simulink model "ar_lht_hw"  (R2018a)
settings: Solver=VariableStepAuto  StartTime=0.0  StopTime=ts*3+maxRho*2*T*3  RelTol=1e-3  EnableMultiTasking=on
PreLoadFcn:
  | currentDir  = pwd;
  | filesepIdx   = strfind(currentDir, filesep);
  | newDir = currentDir(1:filesepIdx(end)-7);
  | 
  | addpath([newDir, '\scripts']);
InitFcn:
  | setup;
  | pre_processing;
StopFcn:
  | post_processing;
  | imtool(O);
values from neighbouring files (symbols this model uses):
  deltaTheta = 1    [setup.m]
  fps = f/((height)*(width))    (= 1475.01627604)    [setup.m]
  height = 256    [setup.m]
  K = (maxTheta + deltaTheta)/R    (= 45)    [setup.m]
  maxRho = ceil(sqrt((height/2)^2+(width/2)^2))    [setup.m]
  maxTheta = 179    [setup.m]
  R = 4    [setup.m]
  T = 1/f    (= 6.89655172414e-09)    [setup.m]
  width = 384    [setup.m]
libraries: xbsIndex_r4 x336, hdlsllib x6, visionhdlutilities x2, visionhdlio x2, simulink x1, dspswit3 x1, visionsources x1
(part 2 of 2)

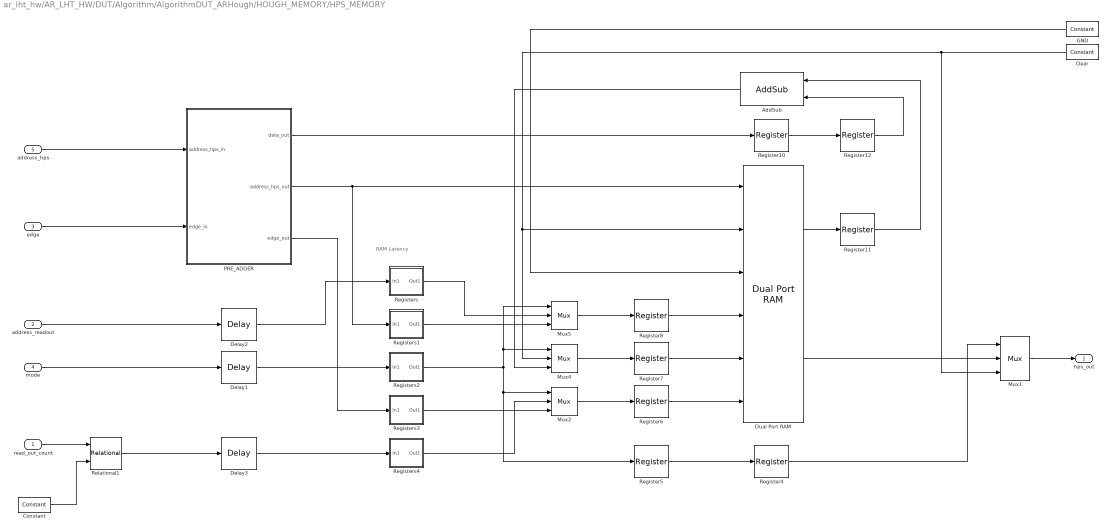
== system ar_lht_hw/AR_LHT_HW/DUT/Algorithm/AlgorithmDUT_ARHough/HOUGH_MEMORY/HPS_MEMORY ==
  note: RAM Latency
  read_out_count : Inport
  address_readout : Inport  Port=2
  edge : Inport  Port=3
  mode : Inport  Port=4
  address_hps : Inport  Port=5
  AddSub : xbsIndex_r4/AddSub  mode=Addition  use_carryin=off  use_carryout=off  en=off  latency=1  precision=User Defined  arith_type=Unsigned  n_bits=ceil(log2(maxRho*2))  bin_pt=0  quantization=Truncate  overflow=Wrap  use_behavioral_HDL=off  hw_selection=Fabric  pipelined=off  dbl_ovrd=off  block_type=addsub
  Clear : xbsIndex_r4/Constant  const=0  gui_display_data_type=Fixed-point  arith_type=Unsigned  n_bits=9  bin_pt=0  preci_type=Single  exp_width=8  frac_width=24  explicit_period=on  period=T  equ=P=C  opselect=C  inp2=PCIN>>17  opr=+  inp1=P  carry=CIN  dbl_ovrd=off  block_type=constant
  Constant : xbsIndex_r4/Constant  const=R-1  gui_display_data_type=Fixed-point  arith_type=Unsigned  n_bits=ceil(log2(R))  bin_pt=0  preci_type=Single  exp_width=8  frac_width=24  explicit_period=on  period=T  equ=P=C  opselect=C  inp2=PCIN>>17  opr=+  inp1=P  carry=CIN  dbl_ovrd=off  block_type=constant
  Delay1 : xbsIndex_r4/Delay  rst=off  infoeditControl=Selection of Reset will increase slice count due to use of real FFs and instead of SRLs  en=off  latency=7  reg_retiming=off  dbl_ovrd=off  block_type=delay
  Delay2 : xbsIndex_r4/Delay  rst=off  infoeditControl=Selection of Reset will increase slice count due to use of real FFs and instead of SRLs  en=off  latency=7  reg_retiming=off  dbl_ovrd=off  block_type=delay
  Delay3 : xbsIndex_r4/Delay  rst=off  infoeditControl=Selection of Reset will increase slice count due to use of real FFs and instead of SRLs  en=off  latency=7  reg_retiming=off  dbl_ovrd=off  block_type=delay
  Dual Port RAM : xbsIndex_r4/Dual Port RAM  depth=K*maxRho*2  initVector=0  distributed_mem=Block RAM  init_a=0  init_b=0  rst_a=off  rst_b=off  en_a=off  en_b=off  latency=1  write_mode_A=Read Before Write  write_mode_B=Read Before Write  optimize=Area  dbl_ovrd=off  block_type=dpram
  GND : xbsIndex_r4/Constant  const=0  gui_display_data_type=Boolean  arith_type=Boolean  n_bits=18  bin_pt=0  preci_type=Single  exp_width=8  frac_width=24  explicit_period=on  period=T  equ=P=C  opselect=C  inp2=PCIN>>17  opr=+  inp1=P  carry=CIN  dbl_ovrd=off  block_type=constant
  Mux1 : xbsIndex_r4/Mux  inputs=2  en=off  latency=1  precision=Full  arith_type=Unsigned  n_bits=16  bin_pt=14  quantization=Truncate  overflow=Wrap  dbl_ovrd=off  block_type=mux
  Mux2 : xbsIndex_r4/Mux  inputs=2  en=off  latency=0  precision=Full  arith_type=Unsigned  n_bits=16  bin_pt=14  quantization=Truncate  overflow=Wrap  dbl_ovrd=off  block_type=mux
  Mux4 : xbsIndex_r4/Mux  inputs=2  en=off  latency=0  precision=Full  arith_type=Unsigned  n_bits=16  bin_pt=14  quantization=Truncate  overflow=Wrap  dbl_ovrd=off  block_type=mux
  Mux5 : xbsIndex_r4/Mux  inputs=2  en=off  latency=0  precision=Full  arith_type=Unsigned  n_bits=16  bin_pt=14  quantization=Truncate  overflow=Wrap  dbl_ovrd=off  block_type=mux
  PRE_ADDER : Subsystem
  Register{4..8,10..12} (8 alike) : xbsIndex_r4/Register  init=0  rst=off  en=off  dbl_ovrd=off  block_type=register
  Registers : Subsystem
  Registers1 : Subsystem
  Registers2 : Subsystem
  Registers3 : Subsystem
  Registers4 : Subsystem
  Relational1 : xbsIndex_r4/Relational  mode=a=b  op_type=Bool  en=off  latency=0  dbl_ovrd=off  block_type=relational
  hps_out : Outport
  wires:
  Register12/1 -> AddSub/2
  Register11/1 -> AddSub/1
  Delay3/1 -> Registers4/1(In1)
  Delay1/1 -> Registers2/1(In1)
  Delay2/1 -> Registers/1(In1)
  Register10/1 -> Register12/1
  Registers1/1(Out1) -> Mux5/3
  Registers/1(Out1) -> Mux5/2
  Registers2/1(Out1) -> Mux4/1, Mux5/1, Mux2/1, Register5/1
  Registers3/1(Out1) -> Mux2/3
  Registers4/1(Out1) -> Mux2/2
  address_readout/1 -> Delay2/1
  Relational1/1 -> Delay3/1
  mode/1 -> Delay1/1
  AddSub/1 -> Mux4/3
  PRE_ADDER/1(data_out) -> Register10/1
  Dual Port RAM/1 -> Register11/1
  PRE_ADDER/3(edge_out) -> Registers3/1(In1)
  PRE_ADDER/2(address_hps_out) -> Dual Port RAM/1, Registers1/1(In1)
  edge/1 -> PRE_ADDER/2(edge_in)
  address_hps/1 -> PRE_ADDER/1(address_hps_in)
  read_out_count/1 -> Relational1/1
  GND/1 -> Dual Port RAM/3
  Register8/1 -> Dual Port RAM/4
  Mux5/1 -> Register8/1
  Mux4/1 -> Register7/1
  Mux2/1 -> Register6/1
  Register7/1 -> Dual Port RAM/5
  Register6/1 -> Dual Port RAM/6
  Register5/1 -> Register4/1
  Dual Port RAM/2 -> Mux1/2
  Clear/1 -> Mux1/3, Mux4/2, Dual Port RAM/2
  Mux1/1 -> hps_out/1
  Constant/1 -> Relational1/2
  Register4/1 -> Mux1/1

== system ar_lht_hw/AR_LHT_HW/DUT/Algorithm/AlgorithmDUT_ARHough/HOUGH_MEMORY/RBM_MEMORY ==
  edge : Inport
  mode : Inport  Port=2
  address_rbm : Inport  Port=3
  readout_rbm : Inport  Port=4
  ClearData : xbsIndex_r4/Constant  const=0  gui_display_data_type=Boolean  arith_type=Boolean  n_bits=9  bin_pt=0  preci_type=Single  exp_width=8  frac_width=24  explicit_period=on  period=T  equ=P=C  opselect=C  inp2=PCIN>>17  opr=+  inp1=P  carry=CIN  dbl_ovrd=off  block_type=constant
  Delay4 : xbsIndex_r4/Delay  rst=off  infoeditControl=Selection of Reset will increase slice count due to use of real FFs and instead of SRLs  en=off  latency=10  reg_retiming=off  dbl_ovrd=off  block_type=delay
  Mux1 : xbsIndex_r4/Mux  inputs=2  en=off  latency=1  precision=User Defined  arith_type=Unsigned  n_bits=1  bin_pt=0  quantization=Truncate  overflow=Wrap  dbl_ovrd=off  block_type=mux
  Mux4 : xbsIndex_r4/Mux  inputs=2  en=off  latency=0  precision=Full  arith_type=Unsigned  n_bits=16  bin_pt=14  quantization=Truncate  overflow=Wrap  dbl_ovrd=off  block_type=mux
  Mux6 : xbsIndex_r4/Mux  inputs=2  en=off  latency=0  precision=Full  arith_type=Unsigned  n_bits=16  bin_pt=14  quantization=Truncate  overflow=Wrap  dbl_ovrd=off  block_type=mux
  Mux7 : xbsIndex_r4/Mux  inputs=2  en=off  latency=0  precision=Full  arith_type=Unsigned  n_bits=16  bin_pt=14  quantization=Truncate  overflow=Wrap  dbl_ovrd=off  block_type=mux
  Register{1..5} (5 alike) : xbsIndex_r4/Register  init=0  rst=off  en=off  dbl_ovrd=off  block_type=register
  Single Port RAM : xbsIndex_r4/Single Port RAM  depth=(maxTheta+deltaTheta)*maxRho*2  initVector=0  distributed_mem=Block RAM  write_mode=Read Before Write  rst=off  init_reg=0  en=off  latency=1  optimize=Area  dbl_ovrd=off  block_type=spram
  vcc : xbsIndex_r4/Constant  const=1  gui_display_data_type=Boolean  arith_type=Boolean  n_bits=9  bin_pt=0  preci_type=Single  exp_width=8  frac_width=24  explicit_period=on  period=T  equ=P=C  opselect=C  inp2=PCIN>>17  opr=+  inp1=P  carry=CIN  dbl_ovrd=off  block_type=constant
  rbm_out : Outport
  wires:
  Delay4/1 -> rbm_out/1
  Register5/1 -> Single Port RAM/1
  Register4/1 -> Single Port RAM/2
  Register3/1 -> Single Port RAM/3
  Register2/1 -> Register1/1
  Register1/1 -> Mux1/1
  mode/1 -> Mux7/1, Mux6/1, Mux4/1, Register2/1
  Single Port RAM/1 -> Mux1/2
  Mux1/1 -> Delay4/1
  vcc/1 -> Mux7/2, Mux6/3
  edge/1 -> Mux7/3
  ClearData/1 -> Mux1/3, Mux6/2
  Mux6/1 -> Register4/1
  Mux7/1 -> Register3/1
  Mux4/1 -> Register5/1
  address_rbm/1 -> Mux4/3
  readout_rbm/1 -> Mux4/2

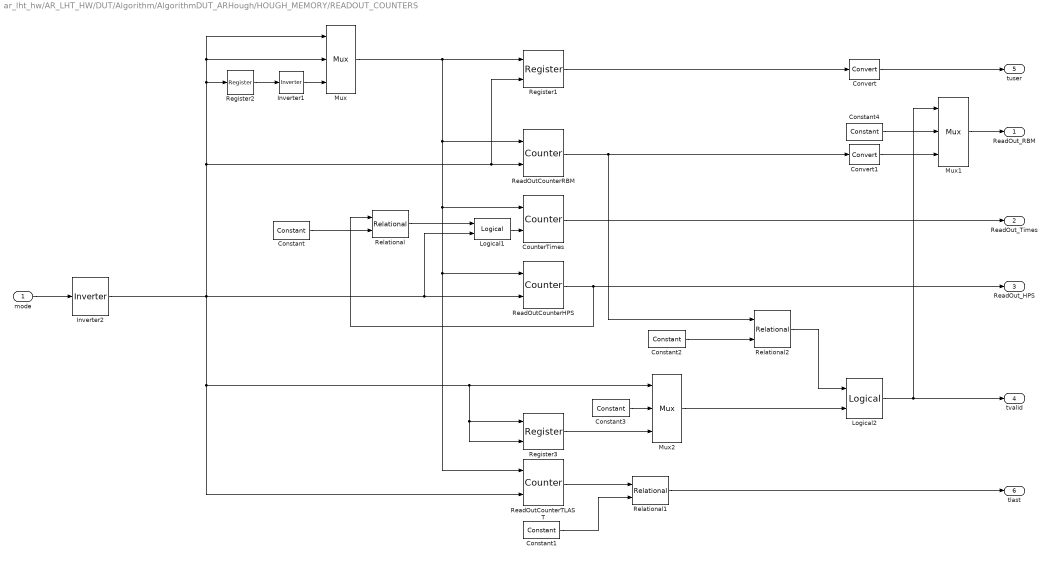
== system ar_lht_hw/AR_LHT_HW/DUT/Algorithm/AlgorithmDUT_ARHough/HOUGH_MEMORY/READOUT_COUNTERS ==
  mode : Inport
  Constant : xbsIndex_r4/Constant  const=K*maxRho*2-2  gui_display_data_type=Fixed-point  arith_type=Unsigned  n_bits=ceil(log2(K*maxRho*2-2))  bin_pt=0  preci_type=Single  exp_width=8  frac_width=24  explicit_period=on  period=T  equ=P=C  opselect=C  inp2=PCIN>>17  opr=+  inp1=P  carry=CIN  dbl_ovrd=off  block_type=constant
  Constant1 : xbsIndex_r4/Constant  const=2*maxRho-1  gui_display_data_type=Fixed-point  arith_type=Unsigned  n_bits=ceil(log2(2*maxRho-1))  bin_pt=0  preci_type=Single  exp_width=8  frac_width=24  explicit_period=on  period=T  equ=P=C  opselect=C  inp2=PCIN>>17  opr=+  inp1=P  carry=CIN  dbl_ovrd=off  block_type=constant
  Constant2 : xbsIndex_r4/Constant  const=(maxTheta+deltaTheta)*maxRho*2-1  gui_display_data_type=Fixed-point  arith_type=Unsigned  n_bits=ceil(log2((maxTheta+deltaTheta)*maxRho*2-1))  bin_pt=0  preci_type=Single  exp_width=8  frac_width=24  explicit_period=on  period=T  equ=P=C  opselect=C  inp2=PCIN>>17  opr=+  inp1=P  carry=CIN  dbl_ovrd=off  block_type=constant
  Constant3 : xbsIndex_r4/Constant  const=0  gui_display_data_type=Boolean  arith_type=Boolean  n_bits=16  bin_pt=14  preci_type=Single  exp_width=8  frac_width=24  explicit_period=on  period=T  equ=P=C  opselect=C  inp2=PCIN>>17  opr=+  inp1=P  carry=CIN  dbl_ovrd=off  block_type=constant
  Constant4 : xbsIndex_r4/Constant  const=0  gui_display_data_type=Fixed-point  arith_type=Unsigned  n_bits=ceil(log2((maxTheta+deltaTheta)*maxRho*2-1))  bin_pt=0  preci_type=Single  exp_width=8  frac_width=24  explicit_period=on  period=T  equ=P=C  opselect=C  inp2=PCIN>>17  opr=+  inp1=P  carry=CIN  dbl_ovrd=off  block_type=constant
  Convert : xbsIndex_r4/Convert  gui_display_data_type=Fixed-point  arith_type=Unsigned  n_bits=1  bin_pt=0  float_type=Single  exp_bits=8  fraction_bits=24  quantization=Truncate  overflow=Wrap  en=off  latency=0  pipeline=off  dbl_ovrd=off  block_type=convert
  Convert1 : xbsIndex_r4/Convert  gui_display_data_type=Fixed-point  arith_type=Unsigned  n_bits=ceil(log2((maxTheta+deltaTheta)*maxRho*2-1))  bin_pt=0  float_type=Single  exp_bits=8  fraction_bits=24  quantization=Truncate  overflow=Wrap  en=off  latency=0  pipeline=off  dbl_ovrd=off  block_type=convert
  CounterTimes : xbsIndex_r4/Counter  cnt_type=Count Limited  cnt_to=R-1  operation=Up  start_count=0  cnt_by_val=1  arith_type=Unsigned  n_bits=ceil(log2(R))  bin_pt=0  load_pin=off  rst=on  en=on  explicit_period=on  period=T  use_behavioral_HDL=on  implementation=Fabric  dbl_ovrd=off  block_type=counter
  Inverter1 : xbsIndex_r4/Inverter  en=off  latency=0  dbl_ovrd=off  block_type=inv
  Inverter2 : xbsIndex_r4/Inverter  en=off  latency=0  dbl_ovrd=off  block_type=inv
  Logical1 : xbsIndex_r4/Logical  logical_function=AND  inputs=2  en=off  latency=0  precision=Full  arith_type=Unsigned  n_bits=16  bin_pt=0  align_bp=on  dbl_ovrd=off  block_type=logical
  Logical2 : xbsIndex_r4/Logical  logical_function=AND  inputs=2  en=off  latency=0  precision=Full  arith_type=Unsigned  n_bits=16  bin_pt=0  align_bp=on  dbl_ovrd=off  block_type=logical
  Mux : xbsIndex_r4/Mux  inputs=2  en=off  latency=0  precision=Full  arith_type=Unsigned  n_bits=16  bin_pt=14  quantization=Truncate  overflow=Wrap  dbl_ovrd=off  block_type=mux
  Mux1 : xbsIndex_r4/Mux  inputs=2  en=off  latency=0  precision=Full  arith_type=Unsigned  n_bits=16  bin_pt=14  quantization=Truncate  overflow=Wrap  dbl_ovrd=off  block_type=mux
  Mux2 : xbsIndex_r4/Mux  inputs=2  en=off  latency=0  precision=Full  arith_type=Unsigned  n_bits=16  bin_pt=14  quantization=Truncate  overflow=Wrap  dbl_ovrd=off  block_type=mux
  ReadOutCounterHPS : xbsIndex_r4/Counter  cnt_type=Count Limited  cnt_to=K*maxRho*2-1  operation=Up  start_count=0  cnt_by_val=1  arith_type=Unsigned  n_bits=ceil(log2(K*maxRho*2-1))  bin_pt=0  load_pin=off  rst=on  en=on  explicit_period=on  period=T  use_behavioral_HDL=on  implementation=Fabric  dbl_ovrd=off  block_type=counter
  ReadOutCounterRBM : xbsIndex_r4/Counter  cnt_type=Free Running  cnt_to=(maxTheta+deltaTheta)*maxRho*2-1  operation=Up  start_count=0  cnt_by_val=1  arith_type=Unsigned  n_bits=32  bin_pt=0  load_pin=off  rst=on  en=on  explicit_period=on  period=T  use_behavioral_HDL=on  implementation=Fabric  dbl_ovrd=off  block_type=counter
  ReadOutCounterTLAST : xbsIndex_r4/Counter  cnt_type=Count Limited  cnt_to=2*maxRho - 1  operation=Up  start_count=0  cnt_by_val=1  arith_type=Unsigned  n_bits=ceil(log2(2*maxRho-1))  bin_pt=0  load_pin=off  rst=on  en=on  explicit_period=on  period=T  use_behavioral_HDL=on  implementation=Fabric  dbl_ovrd=off  block_type=counter
  Register1 : xbsIndex_r4/Register  init=0  rst=off  en=on  dbl_ovrd=off  block_type=register
  Register2 : xbsIndex_r4/Register  init=0  rst=off  en=off  dbl_ovrd=off  block_type=register
  Register3 : xbsIndex_r4/Register  init=0  rst=off  en=on  dbl_ovrd=off  block_type=register
  Relational : xbsIndex_r4/Relational  mode=a=b  op_type=Bool  en=off  latency=1  dbl_ovrd=off  block_type=relational
  Relational1 : xbsIndex_r4/Relational  mode=a=b  op_type=Bool  en=off  latency=0  dbl_ovrd=off  block_type=relational
  Relational2 : xbsIndex_r4/Relational  mode=a<=b  op_type=Bool  en=off  latency=0  dbl_ovrd=off  block_type=relational
  ReadOut_RBM : Outport
  ReadOut_Times : Outport  Port=2
  ReadOut_HPS : Outport  Port=3
  tvalid : Outport  Port=4
  tuser : Outport  Port=5
  tlast : Outport  Port=6
  wires:
  Logical2/1 -> Mux1/1, tvalid/1
  Constant4/1 -> Mux1/2
  Convert1/1 -> Mux1/3
  Mux1/1 -> ReadOut_RBM/1
  Constant3/1 -> Mux2/2
  Inverter2/1 -> Register2/1, Mux/2, Mux/1, ReadOutCounterRBM/2, Register1/2, ReadOutCounterHPS/2, Logical1/2, Mux2/1, Register3/1, Register3/2, ReadOutCounterTLAST/2
  Mux2/1 -> Logical2/2
  Register3/1 -> Mux2/3
  Relational2/1 -> Logical2/1
  Register1/1 -> Convert/1
  Mux/1 -> ReadOutCounterRBM/1, CounterTimes/1, ReadOutCounterHPS/1, ReadOutCounterTLAST/1, Register1/1
  Constant2/1 -> Relational2/2
  Convert/1 -> tuser/1
  Constant1/1 -> Relational1/2
  ReadOutCounterTLAST/1 -> Relational1/1
  Relational1/1 -> tlast/1
  Inverter1/1 -> Mux/3
  Register2/1 -> Inverter1/1
  mode/1 -> Inverter2/1
  ReadOutCounterHPS/1 -> Relational/1, ReadOut_HPS/1
  CounterTimes/1 -> ReadOut_Times/1
  ReadOutCounterRBM/1 -> Convert1/1, Relational2/1
  Constant/1 -> Relational/2
  Logical1/1 -> CounterTimes/2
  Relational/1 -> Logical1/1

== system ar_lht_hw/AR_LHT_HW/DUT/Algorithm/AlgorithmDUT_Open/MorphoOpen/POSITION_CALCULATOR ==
  tuser_in : Inport
  tvalid_in : Inport  Port=2
  Constant1 : xbsIndex_r4/Constant  const=width/2  gui_display_data_type=Fixed-point  arith_type=Unsigned  n_bits=ceil(log2(width/2))+1  bin_pt=0  preci_type=Single  exp_width=8  frac_width=24  explicit_period=on  period=T  equ=P=C  opselect=C  inp2=PCIN>>17  opr=+  inp1=P  carry=CIN  dbl_ovrd=off  block_type=constant
  Constant2 : xbsIndex_r4/Constant  const=height/2  gui_display_data_type=Fixed-point  arith_type=Unsigned  n_bits=ceil(log2(height/2))+1  bin_pt=0  preci_type=Single  exp_width=8  frac_width=24  explicit_period=on  period=T  equ=P=C  opselect=C  inp2=PCIN>>17  opr=+  inp1=P  carry=CIN  dbl_ovrd=off  block_type=constant
  Convert : xbsIndex_r4/Convert  gui_display_data_type=Boolean  arith_type=Boolean  n_bits=16  bin_pt=14  float_type=Single  exp_bits=8  fraction_bits=24  quantization=Truncate  overflow=Wrap  en=off  latency=0  pipeline=off  dbl_ovrd=off  block_type=convert
  Logical : xbsIndex_r4/Logical  logical_function=AND  inputs=2  en=off  latency=0  precision=Full  arith_type=Unsigned  n_bits=16  bin_pt=0  align_bp=on  dbl_ovrd=off  block_type=logical
  Logical1 : xbsIndex_r4/Logical  logical_function=OR  inputs=2  en=off  latency=0  precision=Full  arith_type=Unsigned  n_bits=16  bin_pt=0  align_bp=on  dbl_ovrd=off  block_type=logical
  Logical2 : xbsIndex_r4/Logical  logical_function=AND  inputs=2  en=off  latency=0  precision=Full  arith_type=Unsigned  n_bits=16  bin_pt=0  align_bp=on  dbl_ovrd=off  block_type=logical
  Relational : xbsIndex_r4/Relational  mode=a=b  op_type=Bool  en=off  latency=0  dbl_ovrd=off  block_type=relational
  Relational1 : xbsIndex_r4/Relational  mode=a=b  op_type=Bool  en=off  latency=0  dbl_ovrd=off  block_type=relational
  x_counter : xbsIndex_r4/Counter  cnt_type=Count Limited  cnt_to=width/2  operation=Up  start_count=-width/2+1  cnt_by_val=1  arith_type="Signed  (2's comp)"  n_bits=ceil(log2(width))+1  bin_pt=0  load_pin=off  rst=on  en=on  explicit_period=on  period=T  use_behavioral_HDL=on  implementation=Fabric  dbl_ovrd=off  block_type=counter
  y_counter : xbsIndex_r4/Counter  cnt_type=Count Limited  cnt_to=height/2  operation=Up  start_count=-height/2+1  cnt_by_val=1  arith_type="Signed  (2's comp)"  n_bits=ceil(log2(height))+1  bin_pt=0  load_pin=off  rst=on  en=on  explicit_period=on  period=T  use_behavioral_HDL=on  implementation=Fabric  dbl_ovrd=off  block_type=counter
  x_coordinate : Outport
  y_coordinate : Outport  Port=2
  wires:
  Relational1/1 -> Logical2/2
  Constant2/1 -> Relational1/2
  Logical2/1 -> Logical1/2
  Convert/1 -> Logical1/1
  Logical1/1 -> x_counter/1, y_counter/1
  y_counter/1 -> y_coordinate/1, Relational1/1
  Constant1/1 -> Relational/2
  x_counter/1 -> x_coordinate/1, Relational/1
  tuser_in/1 -> Convert/1
  Logical/1 -> y_counter/2
  Relational/1 -> Logical/1, Logical2/1
  tvalid_in/1 -> Logical/2, x_counter/2

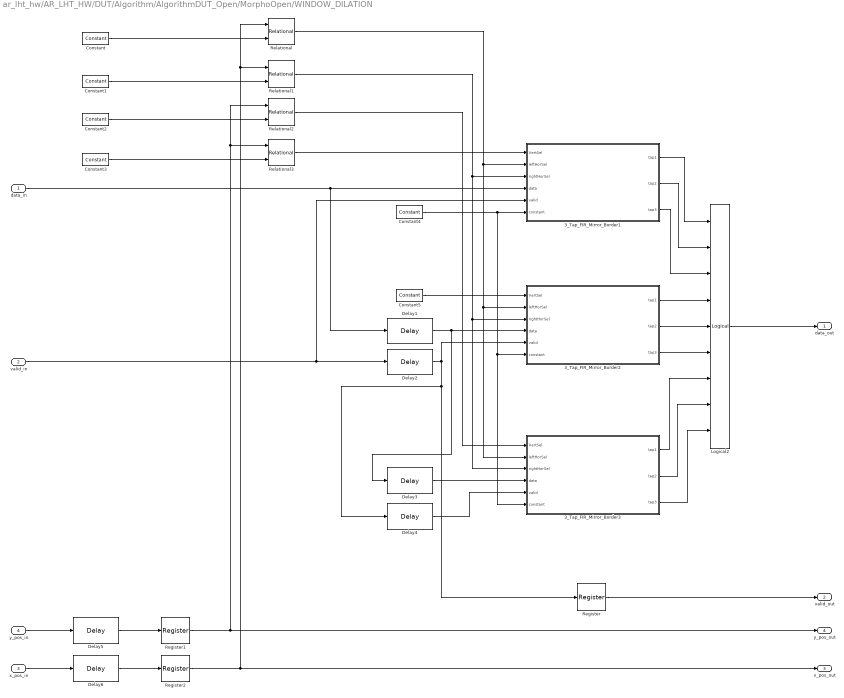
== system ar_lht_hw/AR_LHT_HW/DUT/Algorithm/AlgorithmDUT_Open/MorphoOpen/WINDOW_DILATION ==
  data_in : Inport
  valid_in : Inport  Port=2
  x_pos_in : Inport  Port=3
  y_pos_in : Inport  Port=4
  3_Tap_FIR_Mirror_Border1 : Subsystem
  3_Tap_FIR_Mirror_Border2 : Subsystem
  3_Tap_FIR_Mirror_Border3 : Subsystem
  Constant : xbsIndex_r4/Constant  const=-width/2+1  gui_display_data_type=Fixed-point  arith_type=Signed (2's comp)  n_bits=ceil(log2(width))+1  bin_pt=0  preci_type=Single  exp_width=8  frac_width=24  explicit_period=on  period=T  equ=P=C  opselect=C  inp2=PCIN>>17  opr=+  inp1=P  carry=CIN  dbl_ovrd=off  block_type=constant
  Constant1 : xbsIndex_r4/Constant  const=width/2  gui_display_data_type=Fixed-point  arith_type=Unsigned  n_bits=ceil(log2(width/2))+1  bin_pt=0  preci_type=Single  exp_width=8  frac_width=24  explicit_period=on  period=T  equ=P=C  opselect=C  inp2=PCIN>>17  opr=+  inp1=P  carry=CIN  dbl_ovrd=off  block_type=constant
  Constant2 : xbsIndex_r4/Constant  const=-height/2+1  gui_display_data_type=Fixed-point  arith_type=Signed (2's comp)  n_bits=ceil(log2(height))+1  bin_pt=0  preci_type=Single  exp_width=8  frac_width=24  explicit_period=on  period=T  equ=P=C  opselect=C  inp2=PCIN>>17  opr=+  inp1=P  carry=CIN  dbl_ovrd=off  block_type=constant
  Constant3 : xbsIndex_r4/Constant  const=height/2  gui_display_data_type=Fixed-point  arith_type=Unsigned  n_bits=ceil(log2(height/2))+1  bin_pt=0  preci_type=Single  exp_width=8  frac_width=24  explicit_period=on  period=T  equ=P=C  opselect=C  inp2=PCIN>>17  opr=+  inp1=P  carry=CIN  dbl_ovrd=off  block_type=constant
  Constant4 : xbsIndex_r4/Constant  const=0  gui_display_data_type=Boolean  arith_type=Boolean  n_bits=ceil(log2(width))+1  bin_pt=0  preci_type=Single  exp_width=8  frac_width=24  explicit_period=on  period=T  equ=P=C  opselect=C  inp2=PCIN>>17  opr=+  inp1=P  carry=CIN  dbl_ovrd=off  block_type=constant
  Constant5 : xbsIndex_r4/Constant  const=0  gui_display_data_type=Boolean  arith_type=Boolean  n_bits=ceil(log2(width))+1  bin_pt=0  preci_type=Single  exp_width=8  frac_width=24  explicit_period=on  period=T  equ=P=C  opselect=C  inp2=PCIN>>17  opr=+  inp1=P  carry=CIN  dbl_ovrd=off  block_type=constant
  Delay{1..6} (6 alike) : xbsIndex_r4/Delay  rst=off  infoeditControl=Selection of Reset will increase slice count due to use of real FFs and instead of SRLs  en=off  latency=width  reg_retiming=off  dbl_ovrd=off  block_type=delay
  Logical2 : xbsIndex_r4/Logical  logical_function=OR  inputs=9  en=off  latency=0  precision=Full  arith_type=Unsigned  n_bits=16  bin_pt=0  align_bp=on  dbl_ovrd=off  block_type=logical
  Register : xbsIndex_r4/Register  init=0  rst=off  en=off  dbl_ovrd=off  block_type=register
  Register1 : xbsIndex_r4/Register  init=0  rst=off  en=off  dbl_ovrd=off  block_type=register
  Register2 : xbsIndex_r4/Register  init=0  rst=off  en=off  dbl_ovrd=off  block_type=register
  Relational : xbsIndex_r4/Relational  mode=a<=b  op_type=Bool  en=off  latency=0  dbl_ovrd=off  block_type=relational
  Relational1 : xbsIndex_r4/Relational  mode=a>=b  op_type=Bool  en=off  latency=0  dbl_ovrd=off  block_type=relational
  Relational2 : xbsIndex_r4/Relational  mode=a<=b  op_type=Bool  en=off  latency=0  dbl_ovrd=off  block_type=relational
  Relational3 : xbsIndex_r4/Relational  mode=a>=b  op_type=Bool  en=off  latency=0  dbl_ovrd=off  block_type=relational
  data_out : Outport
  valid_out : Outport  Port=2
  x_pos_out : Outport  Port=3
  y_pos_out : Outport  Port=4
  wires:
  3_Tap_FIR_Mirror_Border3/2(tap2) -> Logical2/8
  3_Tap_FIR_Mirror_Border3/3(tap3) -> Logical2/9
  3_Tap_FIR_Mirror_Border3/1(tap1) -> Logical2/7
  3_Tap_FIR_Mirror_Border2/3(tap3) -> Logical2/6
  3_Tap_FIR_Mirror_Border2/2(tap2) -> Logical2/5
  3_Tap_FIR_Mirror_Border2/1(tap1) -> Logical2/4
  3_Tap_FIR_Mirror_Border1/3(tap3) -> Logical2/3
  3_Tap_FIR_Mirror_Border1/2(tap2) -> Logical2/2
  3_Tap_FIR_Mirror_Border1/1(tap1) -> Logical2/1
  Delay1/1 -> Delay3/1, 3_Tap_FIR_Mirror_Border2/4(data)
  Constant1/1 -> Relational1/2
  Constant3/1 -> Relational3/2
  Constant/1 -> Relational/2
  Constant2/1 -> Relational2/2
  Logical2/1 -> data_out/1
  Constant4/1 -> 3_Tap_FIR_Mirror_Border3/6(constant), 3_Tap_FIR_Mirror_Border2/6(constant), 3_Tap_FIR_Mirror_Border1/6(constant)
  Relational/1 -> 3_Tap_FIR_Mirror_Border3/2(leftHorSel), 3_Tap_FIR_Mirror_Border2/2(leftHorSel), 3_Tap_FIR_Mirror_Border1/2(leftHorSel)
  Delay3/1 -> 3_Tap_FIR_Mirror_Border3/4(data)
  Relational1/1 -> 3_Tap_FIR_Mirror_Border3/3(rightHorSel), 3_Tap_FIR_Mirror_Border2/3(rightHorSel), 3_Tap_FIR_Mirror_Border1/3(rightHorSel)
  Constant5/1 -> 3_Tap_FIR_Mirror_Border2/1(VertSel)
  data_in/1 -> Delay1/1, 3_Tap_FIR_Mirror_Border1/4(data)
  Relational3/1 -> 3_Tap_FIR_Mirror_Border1/1(VertSel)
  Relational2/1 -> 3_Tap_FIR_Mirror_Border3/1(VertSel)
  valid_in/1 -> Delay2/1, 3_Tap_FIR_Mirror_Border1/5(valid)
  Delay5/1 -> Register1/1
  Delay6/1 -> Register2/1
  Delay2/1 -> Delay4/1, Register/1, 3_Tap_FIR_Mirror_Border2/5(valid)
  Delay4/1 -> 3_Tap_FIR_Mirror_Border3/5(valid)
  Register/1 -> valid_out/1
  Register1/1 -> Relational3/1, Relational2/1, y_pos_out/1
  Register2/1 -> Relational1/1, Relational/1, x_pos_out/1
  x_pos_in/1 -> Delay6/1
  y_pos_in/1 -> Delay5/1

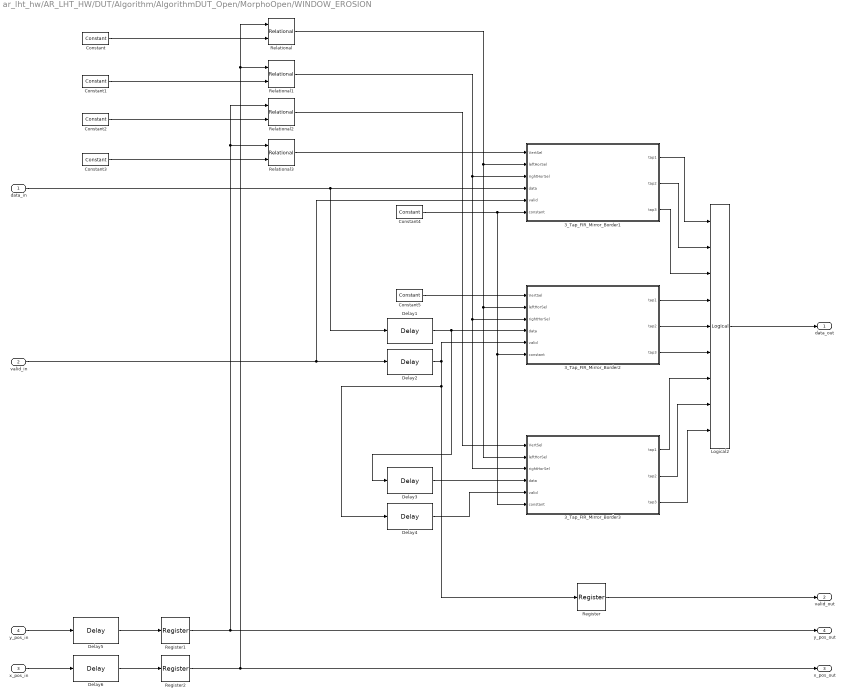
== system ar_lht_hw/AR_LHT_HW/DUT/Algorithm/AlgorithmDUT_Open/MorphoOpen/WINDOW_EROSION ==
  data_in : Inport
  valid_in : Inport  Port=2
  x_pos_in : Inport  Port=3
  y_pos_in : Inport  Port=4
  3_Tap_FIR_Mirror_Border1 : Subsystem
  3_Tap_FIR_Mirror_Border2 : Subsystem
  3_Tap_FIR_Mirror_Border3 : Subsystem
  Constant : xbsIndex_r4/Constant  const=-width/2+1  gui_display_data_type=Fixed-point  arith_type=Signed (2's comp)  n_bits=ceil(log2(width))+1  bin_pt=0  preci_type=Single  exp_width=8  frac_width=24  explicit_period=on  period=T  equ=P=C  opselect=C  inp2=PCIN>>17  opr=+  inp1=P  carry=CIN  dbl_ovrd=off  block_type=constant
  Constant1 : xbsIndex_r4/Constant  const=width/2  gui_display_data_type=Fixed-point  arith_type=Unsigned  n_bits=ceil(log2(width/2))+1  bin_pt=0  preci_type=Single  exp_width=8  frac_width=24  explicit_period=on  period=T  equ=P=C  opselect=C  inp2=PCIN>>17  opr=+  inp1=P  carry=CIN  dbl_ovrd=off  block_type=constant
  Constant2 : xbsIndex_r4/Constant  const=-height/2+1  gui_display_data_type=Fixed-point  arith_type=Signed (2's comp)  n_bits=ceil(log2(height))+1  bin_pt=0  preci_type=Single  exp_width=8  frac_width=24  explicit_period=on  period=T  equ=P=C  opselect=C  inp2=PCIN>>17  opr=+  inp1=P  carry=CIN  dbl_ovrd=off  block_type=constant
  Constant3 : xbsIndex_r4/Constant  const=height/2  gui_display_data_type=Fixed-point  arith_type=Unsigned  n_bits=ceil(log2(height/2))+1  bin_pt=0  preci_type=Single  exp_width=8  frac_width=24  explicit_period=on  period=T  equ=P=C  opselect=C  inp2=PCIN>>17  opr=+  inp1=P  carry=CIN  dbl_ovrd=off  block_type=constant
  Constant4 : xbsIndex_r4/Constant  const=1  gui_display_data_type=Boolean  arith_type=Boolean  n_bits=ceil(log2(width))+1  bin_pt=0  preci_type=Single  exp_width=8  frac_width=24  explicit_period=on  period=T  equ=P=C  opselect=C  inp2=PCIN>>17  opr=+  inp1=P  carry=CIN  dbl_ovrd=off  block_type=constant
  Constant5 : xbsIndex_r4/Constant  const=0  gui_display_data_type=Boolean  arith_type=Boolean  n_bits=ceil(log2(width))+1  bin_pt=0  preci_type=Single  exp_width=8  frac_width=24  explicit_period=on  period=T  equ=P=C  opselect=C  inp2=PCIN>>17  opr=+  inp1=P  carry=CIN  dbl_ovrd=off  block_type=constant
  Delay{1..6} (6 alike) : xbsIndex_r4/Delay  rst=off  infoeditControl=Selection of Reset will increase slice count due to use of real FFs and instead of SRLs  en=off  latency=width  reg_retiming=off  dbl_ovrd=off  block_type=delay
  Logical2 : xbsIndex_r4/Logical  logical_function=AND  inputs=9  en=off  latency=0  precision=Full  arith_type=Unsigned  n_bits=16  bin_pt=0  align_bp=on  dbl_ovrd=off  block_type=logical
  Register : xbsIndex_r4/Register  init=0  rst=off  en=off  dbl_ovrd=off  block_type=register
  Register1 : xbsIndex_r4/Register  init=0  rst=off  en=off  dbl_ovrd=off  block_type=register
  Register2 : xbsIndex_r4/Register  init=0  rst=off  en=off  dbl_ovrd=off  block_type=register
  Relational : xbsIndex_r4/Relational  mode=a<=b  op_type=Bool  en=off  latency=0  dbl_ovrd=off  block_type=relational
  Relational1 : xbsIndex_r4/Relational  mode=a>=b  op_type=Bool  en=off  latency=0  dbl_ovrd=off  block_type=relational
  Relational2 : xbsIndex_r4/Relational  mode=a<=b  op_type=Bool  en=off  latency=0  dbl_ovrd=off  block_type=relational
  Relational3 : xbsIndex_r4/Relational  mode=a>=b  op_type=Bool  en=off  latency=0  dbl_ovrd=off  block_type=relational
  data_out : Outport
  valid_out : Outport  Port=2
  x_pos_out : Outport  Port=3
  y_pos_out : Outport  Port=4
  wires:
  y_pos_in/1 -> Delay5/1
  x_pos_in/1 -> Delay6/1
  Register2/1 -> x_pos_out/1, Relational/1, Relational1/1
  Register1/1 -> y_pos_out/1, Relational2/1, Relational3/1
  Register/1 -> valid_out/1
  Delay4/1 -> 3_Tap_FIR_Mirror_Border3/5(valid)
  Delay2/1 -> 3_Tap_FIR_Mirror_Border2/5(valid), Register/1, Delay4/1
  Delay6/1 -> Register2/1
  Delay5/1 -> Register1/1
  valid_in/1 -> 3_Tap_FIR_Mirror_Border1/5(valid), Delay2/1
  Relational2/1 -> 3_Tap_FIR_Mirror_Border3/1(VertSel)
  Relational3/1 -> 3_Tap_FIR_Mirror_Border1/1(VertSel)
  data_in/1 -> 3_Tap_FIR_Mirror_Border1/4(data), Delay1/1
  Constant5/1 -> 3_Tap_FIR_Mirror_Border2/1(VertSel)
  Relational1/1 -> 3_Tap_FIR_Mirror_Border1/3(rightHorSel), 3_Tap_FIR_Mirror_Border2/3(rightHorSel), 3_Tap_FIR_Mirror_Border3/3(rightHorSel)
  Delay3/1 -> 3_Tap_FIR_Mirror_Border3/4(data)
  Relational/1 -> 3_Tap_FIR_Mirror_Border1/2(leftHorSel), 3_Tap_FIR_Mirror_Border2/2(leftHorSel), 3_Tap_FIR_Mirror_Border3/2(leftHorSel)
  Constant4/1 -> 3_Tap_FIR_Mirror_Border1/6(constant), 3_Tap_FIR_Mirror_Border2/6(constant), 3_Tap_FIR_Mirror_Border3/6(constant)
  Logical2/1 -> data_out/1
  Constant2/1 -> Relational2/2
  Constant/1 -> Relational/2
  Constant3/1 -> Relational3/2
  Constant1/1 -> Relational1/2
  Delay1/1 -> 3_Tap_FIR_Mirror_Border2/4(data), Delay3/1
  3_Tap_FIR_Mirror_Border1/1(tap1) -> Logical2/1
  3_Tap_FIR_Mirror_Border1/2(tap2) -> Logical2/2
  3_Tap_FIR_Mirror_Border1/3(tap3) -> Logical2/3
  3_Tap_FIR_Mirror_Border2/1(tap1) -> Logical2/4
  3_Tap_FIR_Mirror_Border2/2(tap2) -> Logical2/5
  3_Tap_FIR_Mirror_Border2/3(tap3) -> Logical2/6
  3_Tap_FIR_Mirror_Border3/1(tap1) -> Logical2/7
  3_Tap_FIR_Mirror_Border3/3(tap3) -> Logical2/9
  3_Tap_FIR_Mirror_Border3/2(tap2) -> Logical2/8

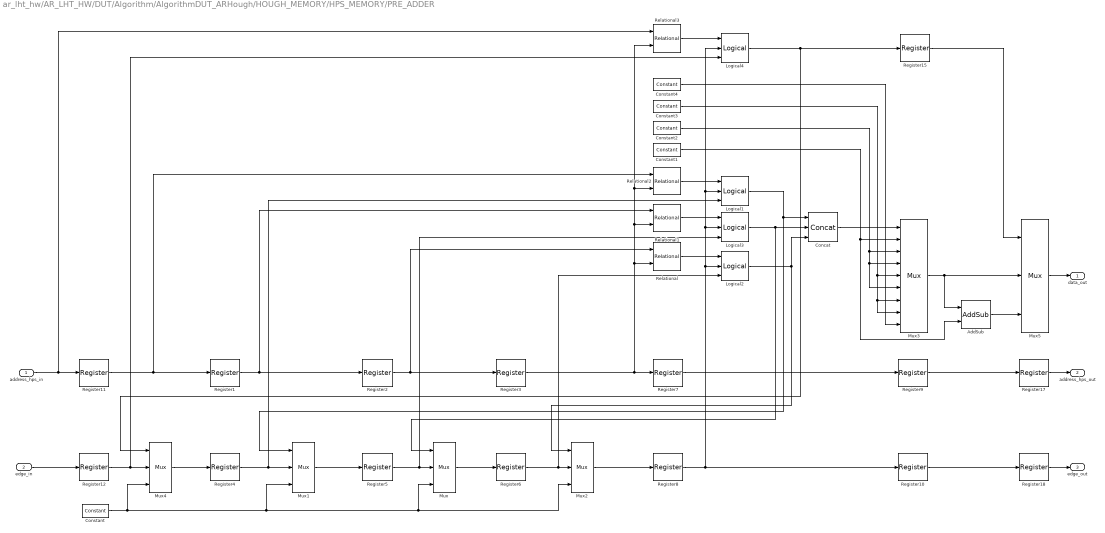
== system ar_lht_hw/AR_LHT_HW/DUT/Algorithm/AlgorithmDUT_ARHough/HOUGH_MEMORY/HPS_MEMORY/PRE_ADDER ==
  address_hps_in : Inport
  edge_in : Inport  Port=2
  AddSub : xbsIndex_r4/AddSub  mode=Addition  use_carryin=off  use_carryout=off  en=off  latency=0  precision=User Defined  arith_type=Unsigned  n_bits=3  bin_pt=0  quantization=Truncate  overflow=Wrap  use_behavioral_HDL=off  hw_selection=Fabric  pipelined=off  dbl_ovrd=off  block_type=addsub
  Concat : xbsIndex_r4/Concat  num_inputs=3  dbl_ovrd=off  block_type=concat
  Constant : xbsIndex_r4/Constant  const=0  gui_display_data_type=Boolean  arith_type=Boolean  n_bits=16  bin_pt=14  preci_type=Single  exp_width=8  frac_width=24  explicit_period=on  period=T  equ=P=C  opselect=C  inp2=PCIN>>17  opr=+  inp1=P  carry=CIN  dbl_ovrd=off  block_type=constant
  Constant1 : xbsIndex_r4/Constant  const=1  gui_display_data_type=Fixed-point  arith_type=Unsigned  n_bits=3  bin_pt=0  preci_type=Single  exp_width=8  frac_width=24  explicit_period=on  period=T  equ=P=C  opselect=C  inp2=PCIN>>17  opr=+  inp1=P  carry=CIN  dbl_ovrd=off  block_type=constant
  Constant2 : xbsIndex_r4/Constant  const=2  gui_display_data_type=Fixed-point  arith_type=Unsigned  n_bits=3  bin_pt=0  preci_type=Single  exp_width=8  frac_width=24  explicit_period=on  period=T  equ=P=C  opselect=C  inp2=PCIN>>17  opr=+  inp1=P  carry=CIN  dbl_ovrd=off  block_type=constant
  Constant3 : xbsIndex_r4/Constant  const=3  gui_display_data_type=Fixed-point  arith_type=Unsigned  n_bits=3  bin_pt=0  preci_type=Single  exp_width=8  frac_width=24  explicit_period=on  period=T  equ=P=C  opselect=C  inp2=PCIN>>17  opr=+  inp1=P  carry=CIN  dbl_ovrd=off  block_type=constant
  Constant4 : xbsIndex_r4/Constant  const=4  gui_display_data_type=Fixed-point  arith_type=Unsigned  n_bits=3  bin_pt=0  preci_type=Single  exp_width=8  frac_width=24  explicit_period=on  period=T  equ=P=C  opselect=C  inp2=PCIN>>17  opr=+  inp1=P  carry=CIN  dbl_ovrd=off  block_type=constant
  Logical{1..4} (4 alike) : xbsIndex_r4/Logical  logical_function=AND  inputs=3  en=off  latency=0  precision=Full  arith_type=Unsigned  n_bits=16  bin_pt=0  align_bp=on  dbl_ovrd=off  block_type=logical
  Mux{,1..2,4} (4 alike) : xbsIndex_r4/Mux  inputs=2  en=off  latency=0  precision=Full  arith_type=Unsigned  n_bits=16  bin_pt=14  quantization=Truncate  overflow=Wrap  dbl_ovrd=off  block_type=mux
  Mux3 : xbsIndex_r4/Mux  inputs=8  en=off  latency=1  precision=Full  arith_type=Unsigned  n_bits=16  bin_pt=14  quantization=Truncate  overflow=Wrap  dbl_ovrd=off  block_type=mux
  Mux5 : xbsIndex_r4/Mux  inputs=2  en=off  latency=1  precision=Full  arith_type=Unsigned  n_bits=16  bin_pt=14  quantization=Truncate  overflow=Wrap  dbl_ovrd=off  block_type=mux
  Register{1..12,15,17..18} (15 alike) : xbsIndex_r4/Register  init=0  rst=off  en=off  dbl_ovrd=off  block_type=register
  Relational{,1..3} (4 alike) : xbsIndex_r4/Relational  mode=a=b  op_type=Bool  en=off  latency=1  dbl_ovrd=off  block_type=relational
  data_out : Outport
  address_hps_out : Outport  Port=2
  edge_out : Outport  Port=3
  wires:
  Register17/1 -> address_hps_out/1
  Register18/1 -> edge_out/1
  Register10/1 -> Register18/1
  Register9/1 -> Register17/1
  Mux5/1 -> data_out/1
  Register15/1 -> Mux5/1
  Logical4/1 -> Register15/1, Mux4/1
  Mux3/1 -> AddSub/1, Mux5/2
  AddSub/1 -> Mux5/3
  Relational3/1 -> Logical4/1
  Mux4/1 -> Register4/1
  Register12/1 -> Logical4/3, Mux4/2
  Register11/1 -> Relational2/1, Register1/1
  Register5/1 -> Mux/2, Logical3/3
  Logical2/1 -> Mux2/1, Concat/3
  Relational/1 -> Logical2/1
  Relational1/1 -> Logical3/1
  Logical3/1 -> Concat/2, Mux/1
  Relational2/1 -> Logical1/1
  Logical1/1 -> Concat/1, Mux1/1
  Constant4/1 -> Mux3/9
  Constant3/1 -> Mux3/5, Mux3/8, Mux3/7
  Constant2/1 -> Mux3/3, Mux3/4, Mux3/6
  Constant1/1 -> Mux3/2, AddSub/2
  Constant/1 -> Mux1/3, Mux2/3, Mux/3, Mux4/3
  Mux2/1 -> Register8/1
  Register6/1 -> Mux2/2, Logical2/3
  Concat/1 -> Mux3/1
  edge_in/1 -> Register12/1
  Register4/1 -> Mux1/2, Logical1/3
  Mux1/1 -> Register5/1
  Mux/1 -> Register6/1
  Register8/1 -> Register10/1, Logical2/2, Logical1/2, Logical4/2, Logical3/2
  Register7/1 -> Register9/1
  Register3/1 -> Relational/2, Relational1/2, Relational2/2, Relational3/2, Register7/1
  Register2/1 -> Relational/1, Register3/1
  Register1/1 -> Relational1/1, Register2/1
  address_hps_in/1 -> Register11/1, Relational3/1

== system ar_lht_hw/AR_LHT_HW/DUT/Algorithm/AlgorithmDUT_ARHough/HOUGH_MEMORY/HPS_MEMORY/Registers ==
  In1 : Inport
  Register1 : xbsIndex_r4/Register  init=0  rst=off  en=off  dbl_ovrd=off  block_type=register
  Register5 : xbsIndex_r4/Register  init=0  rst=off  en=off  dbl_ovrd=off  block_type=register
  Register7 : xbsIndex_r4/Register  init=0  rst=off  en=off  dbl_ovrd=off  block_type=register
  Out1 : Outport
  wires:
  Register1/1 -> Register5/1
  Register7/1 -> Out1/1
  In1/1 -> Register1/1
  Register5/1 -> Register7/1

== system ar_lht_hw/AR_LHT_HW/DUT/Algorithm/AlgorithmDUT_ARHough/HOUGH_MEMORY/HPS_MEMORY/Registers1 ==
  In1 : Inport
  Register1 : xbsIndex_r4/Register  init=0  rst=off  en=off  dbl_ovrd=off  block_type=register
  Register5 : xbsIndex_r4/Register  init=0  rst=off  en=off  dbl_ovrd=off  block_type=register
  Register7 : xbsIndex_r4/Register  init=0  rst=off  en=off  dbl_ovrd=off  block_type=register
  Out1 : Outport
  wires:
  Register5/1 -> Register7/1
  In1/1 -> Register1/1
  Register7/1 -> Out1/1
  Register1/1 -> Register5/1

== system ar_lht_hw/AR_LHT_HW/DUT/Algorithm/AlgorithmDUT_ARHough/HOUGH_MEMORY/HPS_MEMORY/Registers2 ==
  In1 : Inport
  Register1 : xbsIndex_r4/Register  init=0  rst=off  en=off  dbl_ovrd=off  block_type=register
  Register5 : xbsIndex_r4/Register  init=0  rst=off  en=off  dbl_ovrd=off  block_type=register
  Register7 : xbsIndex_r4/Register  init=0  rst=off  en=off  dbl_ovrd=off  block_type=register
  Out1 : Outport
  wires:
  Register1/1 -> Register5/1
  Register7/1 -> Out1/1
  In1/1 -> Register1/1
  Register5/1 -> Register7/1

== system ar_lht_hw/AR_LHT_HW/DUT/Algorithm/AlgorithmDUT_ARHough/HOUGH_MEMORY/HPS_MEMORY/Registers3 ==
  In1 : Inport
  Register1 : xbsIndex_r4/Register  init=0  rst=off  en=off  dbl_ovrd=off  block_type=register
  Register5 : xbsIndex_r4/Register  init=0  rst=off  en=off  dbl_ovrd=off  block_type=register
  Register7 : xbsIndex_r4/Register  init=0  rst=off  en=off  dbl_ovrd=off  block_type=register
  Out1 : Outport
  wires:
  Register5/1 -> Register7/1
  In1/1 -> Register1/1
  Register7/1 -> Out1/1
  Register1/1 -> Register5/1

== system ar_lht_hw/AR_LHT_HW/DUT/Algorithm/AlgorithmDUT_ARHough/HOUGH_MEMORY/HPS_MEMORY/Registers4 ==
  In1 : Inport
  Register1 : xbsIndex_r4/Register  init=0  rst=off  en=off  dbl_ovrd=off  block_type=register
  Register5 : xbsIndex_r4/Register  init=0  rst=off  en=off  dbl_ovrd=off  block_type=register
  Register7 : xbsIndex_r4/Register  init=0  rst=off  en=off  dbl_ovrd=off  block_type=register
  Out1 : Outport
  wires:
  Register1/1 -> Register5/1
  Register7/1 -> Out1/1
  In1/1 -> Register1/1
  Register5/1 -> Register7/1

== system ar_lht_hw/AR_LHT_HW/DUT/Algorithm/AlgorithmDUT_Open/MorphoOpen/WINDOW_DILATION/3_Tap_FIR_Mirror_Border1 ==
  VertSel : Inport
  leftHorSel : Inport  Port=2
  rightHorSel : Inport  Port=3
  data : Inport  Port=4
  valid : Inport  Port=5
  constant : Inport  Port=6
  Mux{,1..4} (5 alike) : xbsIndex_r4/Mux  inputs=2  en=off  latency=0  precision=Full  arith_type=Unsigned  n_bits=16  bin_pt=14  quantization=Truncate  overflow=Wrap  dbl_ovrd=off  block_type=mux
  Register8 : xbsIndex_r4/Register  init=0  rst=off  en=on  dbl_ovrd=off  block_type=register
  Register9 : xbsIndex_r4/Register  init=0  rst=off  en=on  dbl_ovrd=off  block_type=register
  tap1 : Outport
  tap2 : Outport  Port=2
  tap3 : Outport  Port=3
  wires:
  valid/1 -> Register8/2, Register9/2
  Register8/1 -> Mux/2, Register9/1
  data/1 -> Mux3/2, Register8/1
  Mux/1 -> tap2/1
  Mux1/1 -> tap1/1
  Mux2/1 -> tap3/1
  VertSel/1 -> Mux1/1, Mux/1, Mux2/1
  Mux3/1 -> Mux1/2
  Mux4/1 -> Mux2/2
  Register9/1 -> Mux4/2
  constant/1 -> Mux1/3, Mux/3, Mux2/3, Mux3/3, Mux4/3
  leftHorSel/1 -> Mux4/1
  rightHorSel/1 -> Mux3/1

== system ar_lht_hw/AR_LHT_HW/DUT/Algorithm/AlgorithmDUT_Open/MorphoOpen/WINDOW_DILATION/3_Tap_FIR_Mirror_Border2 ==
  VertSel : Inport
  leftHorSel : Inport  Port=2
  rightHorSel : Inport  Port=3
  data : Inport  Port=4
  valid : Inport  Port=5
  constant : Inport  Port=6
  Mux{,1..4} (5 alike) : xbsIndex_r4/Mux  inputs=2  en=off  latency=0  precision=Full  arith_type=Unsigned  n_bits=16  bin_pt=14  quantization=Truncate  overflow=Wrap  dbl_ovrd=off  block_type=mux
  Register8 : xbsIndex_r4/Register  init=0  rst=off  en=on  dbl_ovrd=off  block_type=register
  Register9 : xbsIndex_r4/Register  init=0  rst=off  en=on  dbl_ovrd=off  block_type=register
  tap1 : Outport
  tap2 : Outport  Port=2
  tap3 : Outport  Port=3
  wires:
  rightHorSel/1 -> Mux3/1
  leftHorSel/1 -> Mux4/1
  constant/1 -> Mux4/3, Mux3/3, Mux2/3, Mux/3, Mux1/3
  Register9/1 -> Mux4/2
  Mux4/1 -> Mux2/2
  Mux3/1 -> Mux1/2
  VertSel/1 -> Mux2/1, Mux/1, Mux1/1
  Mux2/1 -> tap3/1
  Mux1/1 -> tap1/1
  Mux/1 -> tap2/1
  data/1 -> Register8/1, Mux3/2
  Register8/1 -> Register9/1, Mux/2
  valid/1 -> Register9/2, Register8/2

== system ar_lht_hw/AR_LHT_HW/DUT/Algorithm/AlgorithmDUT_Open/MorphoOpen/WINDOW_DILATION/3_Tap_FIR_Mirror_Border3 ==
  VertSel : Inport
  leftHorSel : Inport  Port=2
  rightHorSel : Inport  Port=3
  data : Inport  Port=4
  valid : Inport  Port=5
  constant : Inport  Port=6
  Mux{,1..4} (5 alike) : xbsIndex_r4/Mux  inputs=2  en=off  latency=0  precision=Full  arith_type=Unsigned  n_bits=16  bin_pt=14  quantization=Truncate  overflow=Wrap  dbl_ovrd=off  block_type=mux
  Register8 : xbsIndex_r4/Register  init=0  rst=off  en=on  dbl_ovrd=off  block_type=register
  Register9 : xbsIndex_r4/Register  init=0  rst=off  en=on  dbl_ovrd=off  block_type=register
  tap1 : Outport
  tap2 : Outport  Port=2
  tap3 : Outport  Port=3
  wires:
  valid/1 -> Register8/2, Register9/2
  Register8/1 -> Mux/2, Register9/1
  data/1 -> Mux3/2, Register8/1
  Mux/1 -> tap2/1
  Mux1/1 -> tap1/1
  Mux2/1 -> tap3/1
  VertSel/1 -> Mux1/1, Mux/1, Mux2/1
  Mux3/1 -> Mux1/2
  Mux4/1 -> Mux2/2
  Register9/1 -> Mux4/2
  constant/1 -> Mux1/3, Mux/3, Mux2/3, Mux3/3, Mux4/3
  leftHorSel/1 -> Mux4/1
  rightHorSel/1 -> Mux3/1

== system ar_lht_hw/AR_LHT_HW/DUT/Algorithm/AlgorithmDUT_Open/MorphoOpen/WINDOW_EROSION/3_Tap_FIR_Mirror_Border1 ==
  VertSel : Inport
  leftHorSel : Inport  Port=2
  rightHorSel : Inport  Port=3
  data : Inport  Port=4
  valid : Inport  Port=5
  constant : Inport  Port=6
  Mux{,1..4} (5 alike) : xbsIndex_r4/Mux  inputs=2  en=off  latency=0  precision=Full  arith_type=Unsigned  n_bits=16  bin_pt=14  quantization=Truncate  overflow=Wrap  dbl_ovrd=off  block_type=mux
  Register8 : xbsIndex_r4/Register  init=0  rst=off  en=on  dbl_ovrd=off  block_type=register
  Register9 : xbsIndex_r4/Register  init=0  rst=off  en=on  dbl_ovrd=off  block_type=register
  tap1 : Outport
  tap2 : Outport  Port=2
  tap3 : Outport  Port=3
  wires:
  rightHorSel/1 -> Mux3/1
  leftHorSel/1 -> Mux4/1
  constant/1 -> Mux4/3, Mux3/3, Mux2/3, Mux/3, Mux1/3
  Register9/1 -> Mux4/2
  Mux4/1 -> Mux2/2
  Mux3/1 -> Mux1/2
  VertSel/1 -> Mux2/1, Mux/1, Mux1/1
  Mux2/1 -> tap3/1
  Mux1/1 -> tap1/1
  Mux/1 -> tap2/1
  data/1 -> Register8/1, Mux3/2
  Register8/1 -> Register9/1, Mux/2
  valid/1 -> Register9/2, Register8/2

== system ar_lht_hw/AR_LHT_HW/DUT/Algorithm/AlgorithmDUT_Open/MorphoOpen/WINDOW_EROSION/3_Tap_FIR_Mirror_Border2 ==
  VertSel : Inport
  leftHorSel : Inport  Port=2
  rightHorSel : Inport  Port=3
  data : Inport  Port=4
  valid : Inport  Port=5
  constant : Inport  Port=6
  Mux{,1..4} (5 alike) : xbsIndex_r4/Mux  inputs=2  en=off  latency=0  precision=Full  arith_type=Unsigned  n_bits=16  bin_pt=14  quantization=Truncate  overflow=Wrap  dbl_ovrd=off  block_type=mux
  Register8 : xbsIndex_r4/Register  init=0  rst=off  en=on  dbl_ovrd=off  block_type=register
  Register9 : xbsIndex_r4/Register  init=0  rst=off  en=on  dbl_ovrd=off  block_type=register
  tap1 : Outport
  tap2 : Outport  Port=2
  tap3 : Outport  Port=3
  wires:
  valid/1 -> Register8/2, Register9/2
  Register8/1 -> Mux/2, Register9/1
  data/1 -> Mux3/2, Register8/1
  Mux/1 -> tap2/1
  Mux1/1 -> tap1/1
  Mux2/1 -> tap3/1
  VertSel/1 -> Mux1/1, Mux/1, Mux2/1
  Mux3/1 -> Mux1/2
  Mux4/1 -> Mux2/2
  Register9/1 -> Mux4/2
  constant/1 -> Mux1/3, Mux/3, Mux2/3, Mux3/3, Mux4/3
  leftHorSel/1 -> Mux4/1
  rightHorSel/1 -> Mux3/1

== system ar_lht_hw/AR_LHT_HW/DUT/Algorithm/AlgorithmDUT_Open/MorphoOpen/WINDOW_EROSION/3_Tap_FIR_Mirror_Border3 ==
  VertSel : Inport
  leftHorSel : Inport  Port=2
  rightHorSel : Inport  Port=3
  data : Inport  Port=4
  valid : Inport  Port=5
  constant : Inport  Port=6
  Mux{,1..4} (5 alike) : xbsIndex_r4/Mux  inputs=2  en=off  latency=0  precision=Full  arith_type=Unsigned  n_bits=16  bin_pt=14  quantization=Truncate  overflow=Wrap  dbl_ovrd=off  block_type=mux
  Register8 : xbsIndex_r4/Register  init=0  rst=off  en=on  dbl_ovrd=off  block_type=register
  Register9 : xbsIndex_r4/Register  init=0  rst=off  en=on  dbl_ovrd=off  block_type=register
  tap1 : Outport
  tap2 : Outport  Port=2
  tap3 : Outport  Port=3
  wires:
  rightHorSel/1 -> Mux3/1
  leftHorSel/1 -> Mux4/1
  constant/1 -> Mux4/3, Mux3/3, Mux2/3, Mux/3, Mux1/3
  Register9/1 -> Mux4/2
  Mux4/1 -> Mux2/2
  Mux3/1 -> Mux1/2
  VertSel/1 -> Mux2/1, Mux/1, Mux1/1
  Mux2/1 -> tap3/1
  Mux1/1 -> tap1/1
  Mux/1 -> tap2/1
  data/1 -> Register8/1, Mux3/2
  Register8/1 -> Register9/1, Mux/2
  valid/1 -> Register9/2, Register8/2
